simulink model "BirdHeadModel3"  (R2023a)
settings: Solver=FixedStepAuto  StartTime=0.0  StopTime=tsim  FixedStep=dt  RelTol=1e-3
values from neighbouring files (symbols this model uses):
  dt = 0.002    [LaunchBirdHeadModel2.m]    (also in LaunchBirdHeadModelControlled.m; LaunchBirdHeadModelControlled_MovementControl.m; PlotMovementControl.m; PlotPositionControl.m)
  g = 9.81    [LaunchBirdHeadModel2.m]    (also in LaunchBirdHeadModelControlled.m; LaunchBirdHeadModelControlled_MovementControl.m; PlotMovementControl.m; PlotPositionControl.m)
  I_by = 0.00001    (= 1e-05)    [LaunchBirdHeadModel2.m]    (also in LaunchBirdHeadModelControlled.m; LaunchBirdHeadModelControlled_MovementControl.m; PlotMovementControl.m; PlotPositionControl.m)
  I_hy = 0.00001    (= 1e-05)    [LaunchBirdHeadModel2.m]    (also in LaunchBirdHeadModelControlled.m; LaunchBirdHeadModelControlled_MovementControl.m; PlotMovementControl.m; PlotPositionControl.m)
  Kp = [20  0; 0  20]    [CondIni-1010Kp201Kv101.mat]    (also in Kp101Kv51.mat = [20  0; 0  1]; Kp11Kv051.mat = [1  0; 0  1]; Kp11Kv11.mat = [1  0; 0  1]; Kp11Kv21.mat = [1  0; 0  1])
  Kv = [10  0; 0  10]    [CondIni-1010Kp201Kv101.mat]    (also in Kp101Kv51.mat = [5  0; 0  1]; Kp11Kv051.mat = [0.5  0; 0  1]; Kp11Kv11.mat = [1  0; 0  1]; Kp11Kv21.mat = [2  0; 0  1])
  l_b = 0.05    [LaunchBirdHeadModel2.m]    (also in LaunchBirdHeadModelControlled.m; LaunchBirdHeadModelControlled_MovementControl.m; PlotMovementControl.m; PlotPositionControl.m)
  l_h = 0.04    [LaunchBirdHeadModel2.m]    (also in LaunchBirdHeadModelControlled.m; LaunchBirdHeadModelControlled_MovementControl.m; PlotMovementControl.m; PlotPositionControl.m)
  m_h = 0.005    [LaunchBirdHeadModel2.m]    (also in LaunchBirdHeadModelControlled.m; LaunchBirdHeadModelControlled_MovementControl.m; PlotMovementControl.m; PlotPositionControl.m)
settings Model: Creator=coquet  LastModifiedBy=coquet

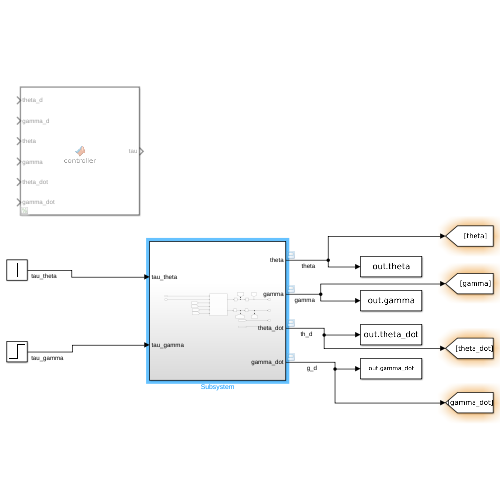
[thumbnail: Simulink's stored preview of the top-level diagram]
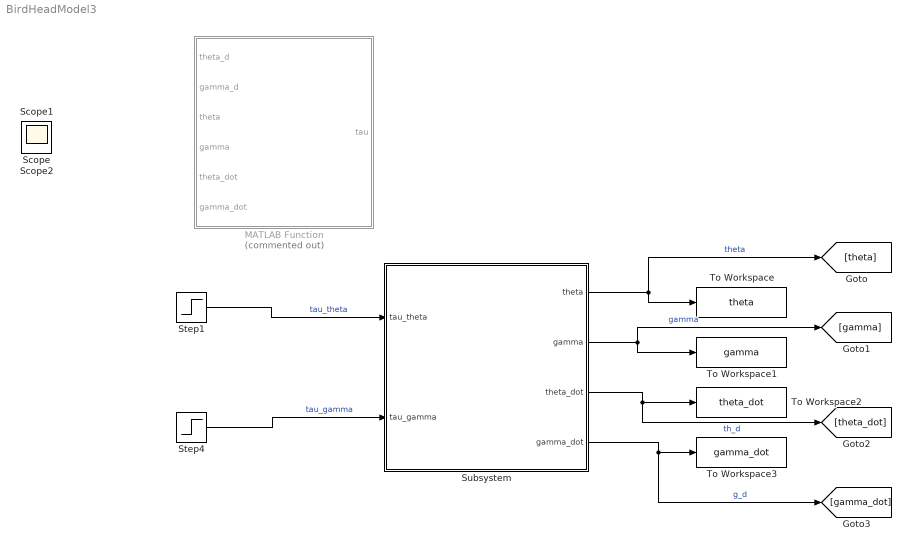
== system BirdHeadModel3 ==
  MATLAB Function : MATLAB Function  Commented=on  TreatAsAtomicUnit=on
  Step1 : Step  After=0  SampleTime=dt
  Step4 : Step  After=0  SampleTime=dt
  Subsystem : Subsystem
  To Workspace : ToWorkspace  VariableName=theta  SaveFormat=Timeseries  SampleTime=dt
  To Workspace1 : ToWorkspace  VariableName=gamma  SaveFormat=Timeseries  SampleTime=dt
  To Workspace2 : ToWorkspace  VariableName=theta_dot  SaveFormat=Timeseries  SampleTime=dt
  To Workspace3 : ToWorkspace  VariableName=gamma_dot  SaveFormat=Timeseries  SampleTime=dt
  Scope : Scope
  Scope1 : Scope
  Scope2 : Scope
  wires:
  Subsystem/4(gamma_dot) -> [gamma_dot], To Workspace3/1  "g_d"
  Subsystem/1(theta) -> To Workspace/1, [theta]  "theta"
  Subsystem/3(theta_dot) -> To Workspace2/1, [theta_dot]  "th_d"
  Subsystem/2(gamma) -> To Workspace1/1, [gamma]  "gamma"
  Step1/1 -> Subsystem/1(tau_theta)  "tau_theta"
  Step4/1 -> Subsystem/2(tau_gamma)  "tau_gamma"

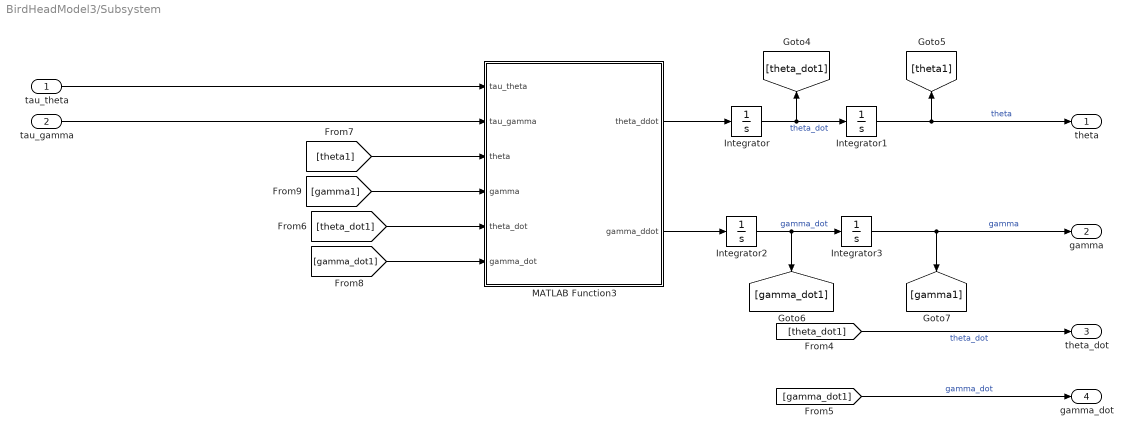
== system BirdHeadModel3/Subsystem ==
  tau_theta : Inport
  tau_gamma : Inport  Port=2
  Integrator : Integrator  ContinuousStateAttributes='theta_dot'
  Integrator1 : Integrator  UpperSaturationLimit=2*pi/9  LowerSaturationLimit=-pi/3  WrapState=on  ContinuousStateAttributes='theta'
  Integrator2 : Integrator  ContinuousStateAttributes='gamma_dot'
  Integrator3 : Integrator  UpperSaturationLimit=2*pi/9  LowerSaturationLimit=-pi/3  WrapState=on  ContinuousStateAttributes='gamma'
  MATLAB Function3 : MATLAB Function  TreatAsAtomicUnit=on
  theta : Outport
  gamma : Outport  Port=2
  theta_dot : Outport  Port=3
  gamma_dot : Outport  Port=4
  wires:
  [gamma1] -> MATLAB Function3/4(gamma)
  Integrator1/1 -> theta/1, [theta1]  "theta"
  [theta1] -> MATLAB Function3/3(theta)
  tau_theta/1 -> MATLAB Function3/1(tau_theta)
  [theta_dot1] -> MATLAB Function3/5(theta_dot)
  MATLAB Function3/1(theta_ddot) -> Integrator/1
  [gamma_dot1] -> MATLAB Function3/6(gamma_dot)
  [theta_dot1] -> theta_dot/1  "theta_dot"
  MATLAB Function3/2(gamma_ddot) -> Integrator2/1
  Integrator3/1 -> gamma/1, [gamma1]  "gamma"
  tau_gamma/1 -> MATLAB Function3/2(tau_gamma)
  Integrator2/1 -> [gamma_dot1], Integrator3/1  "gamma_dot"
  [gamma_dot1] -> gamma_dot/1  "gamma_dot"
  Integrator/1 -> Integrator1/1, [theta_dot1]  "theta_dot"

== matlab function BirdHeadModel3/MATLAB Function ==
  data: tau output; theta_d input; gamma_d input; theta input; gamma input; theta_dot input; gamma_dot input; Kv parameter; Kp parameter
function tau  = controller(theta_d, gamma_d, theta, gamma, theta_dot, gamma_dot, Kv, Kp)

tau = MKp*[theta_d-theta;gamma_d-gamma]-Kv*[theta_dot;gamma_dot];

== matlab function BirdHeadModel3/Subsystem/MATLAB Function3 ==
  data: tau_theta input; tau_gamma input; theta_ddot output; theta input; gamma input; theta_dot input; gamma_dot input; gamma_ddot output; I_hy parameter; m_h parameter; l_b parameter; l_h parameter; I_by parameter; g parameter
function [theta_ddot, gamma_ddot] = fcn(tau_theta, tau_gamma,theta,gamma,theta_dot,gamma_dot, I_hy, m_h, l_b, l_h, I_by,g)

tau = [tau_theta;tau_gamma];

m11 = I_hy+I_by+m_h*(l_b^2+l_h^2)+2*l_b*l_h*m_h*cos(gamma);
m12 = I_hy+m_h*l_h^2+l_b*l_h*m_h*cos(gamma);
m22 = I_hy + l_h^2*m_h;

M=[m11 m12;
   m12 m22];


c11 = -l_b*l_h*m_h*sin(gamma)*gamma_dot;
c12 = -(gamma_dot+theta_dot)*l_b*l_h*m_h*sin(gamma);
c21 = l_b*l_h*m_h*sin(gamma)*theta_dot;
c22 = 0;

C=[c11 c12; 
   c21 c22];

g1 = -g*m_h*cos(theta)*(l_b+l_h*cos(gamma))+g*l_h*m_h*sin(gamma)*sin(theta);
g2 = -l_h*m_h*cos(gamma+theta)*g;

G=[g1;g2];

qddot=M\(tau-C*[theta_dot;gamma_dot]-G);

theta_ddot=qddot(1);
gamma_ddot=qddot(2);
